simulink model "twoPhaseStickmanRev2022a"  (R2022a)
settings: Solver=VariableStepAuto  StartTime=0.0  StopTime=10  RelTol=1e-3
libraries: aerolibanim x1, shared6dof x1
settings Model: Creator=matho  LastModifiedBy=matho
settings ModelReferenceCC: EnableRefExpFcnMdlSchedulingChecks=off
settings RTWCC: Description=Generic Real-Time Target

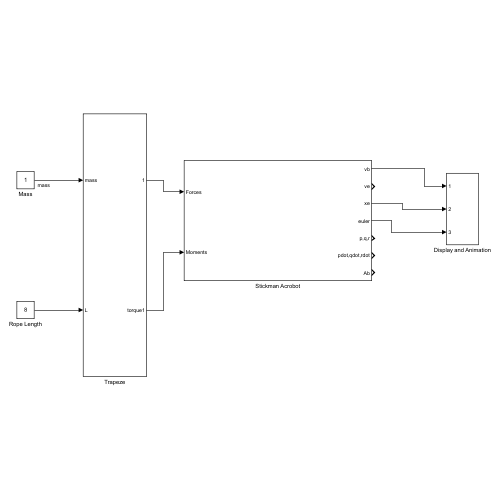
[thumbnail: Simulink's stored preview of the top-level diagram]
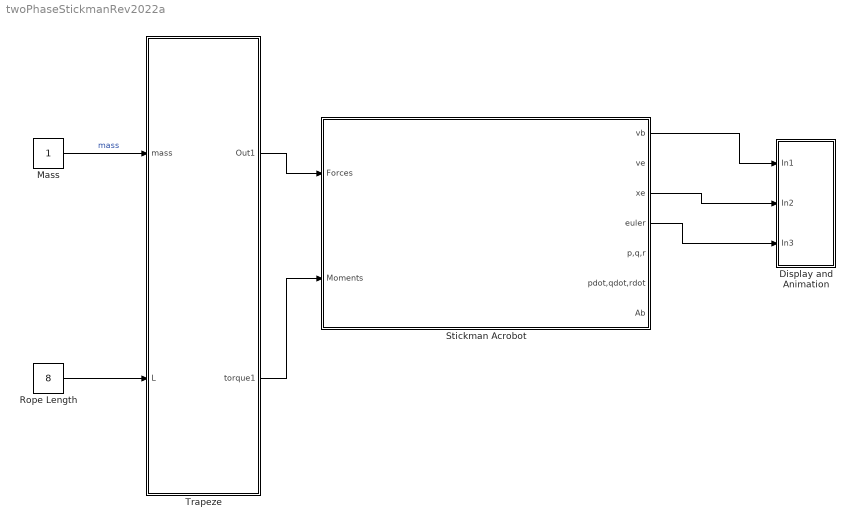
== system twoPhaseStickmanRev2022a ==
  Display and Animation : Subsystem
  Mass : Constant
  Rope Length : Constant  Value=8
  Stickman Acrobot : Subsystem
  Trapeze : Subsystem
  wires:
  Mass/1 -> Trapeze/1(mass)  "mass"
  Rope Length/1 -> Trapeze/2(L)
  Trapeze/1(Out1) -> Stickman Acrobot/1(Forces)
  Trapeze/2(torque1) -> Stickman Acrobot/2(Moments)
  Stickman Acrobot/1(vb) -> Display and Animation/1(In1)
  Stickman Acrobot/3(xe) -> Display and Animation/2(In2)
  Stickman Acrobot/4(euler) -> Display and Animation/3(In3)

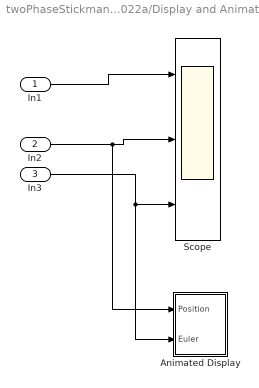
== system twoPhaseStickmanRev2022a/Display and Animation ==
  In1 : Inport
  In2 : Inport  Port=2
  In3 : Inport  Port=3
  Animated Display : Subsystem
  Scope : Scope  NumInputPorts=3
  wires:
  In2/1 -> Animated Display/1(Position), Scope/2
  In3/1 -> Animated Display/2(Euler), Scope/3
  In1/1 -> Scope/1

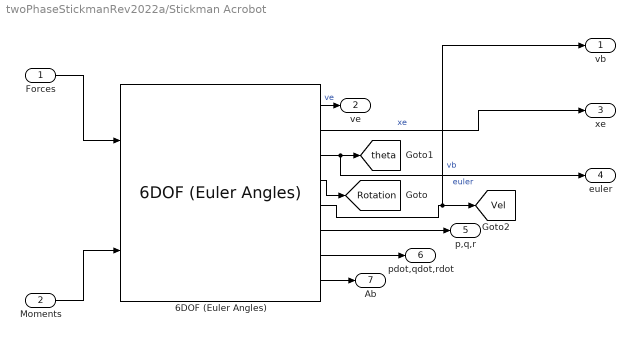
== system twoPhaseStickmanRev2022a/Stickman Acrobot ==
  Forces : Inport
  Moments : Inport  Port=2
  6DOF (Euler Angles) : shared6dof/6DOF (Euler Angles)  units=Metric (MKS)  mtype=Fixed  rep=Euler Angles  xme_0=[-8 0 -8]  Vm_0=[0 0 0]  eul_0=[0 -1.5 0]  pm_0=[0 0 0]  mass_0=1.0  mass_e=0.5  mass_f=2.0  inertia=eye(3)  inertia_e=eye(3)  inertia_f=2*eye(3)  k_quat=1.0  vre_flag=on  abi_flag=off  aMode=0  xme_statename=''  Vm_statename=''  eul_statename=''  quat_statename=''  pm_statename=''  mass_statename=''
  vb : Outport
  ve : Outport  Port=2
  xe : Outport  Port=3
  euler : Outport  Port=4
  p,q,r : Outport  Port=5
  pdot,qdot,rdot : Outport  Port=6
  Ab : Outport  Port=7
  tag scope: Rotation=global, Vel=global, theta=global
  wires:
  Moments/1 -> 6DOF (Euler Angles)/2
  6DOF (Euler Angles)/5 -> vb/1, [Vel]  "vb"
  6DOF (Euler Angles)/3 -> euler/1, [theta]  "euler"
  6DOF (Euler Angles)/8 -> Ab/1
  6DOF (Euler Angles)/4 -> [Rotation]
  6DOF (Euler Angles)/2 -> xe/1  "xe"
  Forces/1 -> 6DOF (Euler Angles)/1
  6DOF (Euler Angles)/6 -> p,q,r/1
  6DOF (Euler Angles)/1 -> ve/1  "ve"
  6DOF (Euler Angles)/7 -> pdot,qdot,rdot/1

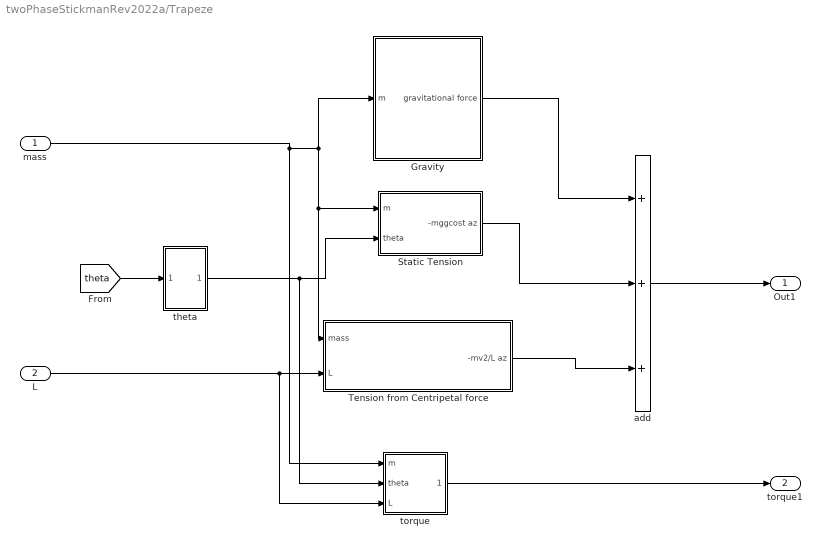
== system twoPhaseStickmanRev2022a/Trapeze ==
  mass : Inport
  L : Inport  Port=2
  Gravity : Subsystem
  Static Tension : Subsystem
  Tension from Centripetal force : Subsystem
  add : Sum  Inputs=+++
  theta : Subsystem
  torque : Subsystem
  Out1 : Outport
  torque1 : Outport  Port=2
  wires:
  theta/1(Out1) -> torque/2(theta), Static Tension/2(theta)
  [theta] -> theta/1(In1)
  mass/1 -> Tension from Centripetal force/1(mass), Static Tension/1(m), Gravity/1(m), torque/1(m)
  Tension from Centripetal force/1(-mv2/L az) -> add/3
  Static Tension/1(-mggcost az) -> add/2
  Gravity/1(gravitational force) -> add/1
  L/1 -> torque/3(L), Tension from Centripetal force/2(L)
  add/1 -> Out1/1
  torque/1(torque) -> torque1/1

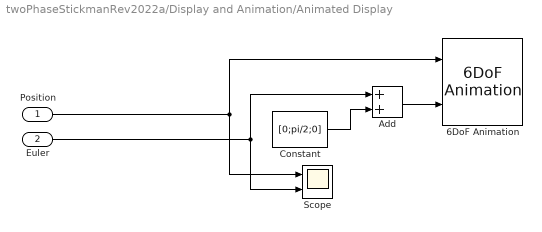
== system twoPhaseStickmanRev2022a/Display and Animation/Animated Display ==
  Position : Inport
  Euler : Inport  Port=2
  6DoF Animation : aerolibanim/6DoF Animation  u1=[-50 50 -50 50 -100 0]  u2=0.05  u3=3.0  u4=[0,0,0]  u5=Fixed position  u6=[10,10,0]  u7=90  u8=on
  Add : Sum
  Constant : Constant  Value=[0;pi/2;0]
  Scope : Scope  NumInputPorts=2
  wires:
  Euler/1 -> Add/1, Scope/2
  Position/1 -> Scope/1, 6DoF Animation/1
  Add/1 -> 6DoF Animation/2
  Constant/1 -> Add/2

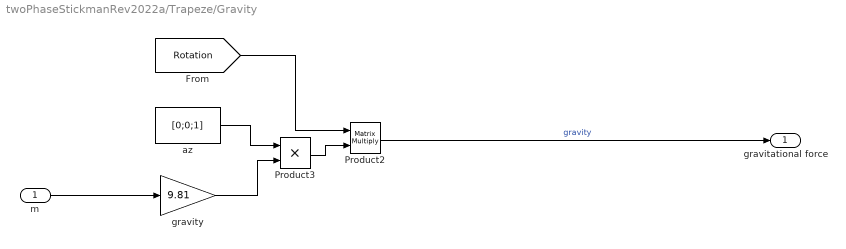
== system twoPhaseStickmanRev2022a/Trapeze/Gravity ==
  m : Inport
  Product2 : Product  Multiplication=Matrix(*)
  Product3 : Product
  az : Constant  Value=[0;0;1]
  gravity : Gain  Gain=9.81
  gravitational force : Outport
  wires:
  [Rotation] -> Product2/1
  az/1 -> Product3/1
  gravity/1 -> Product3/2
  Product3/1 -> Product2/2
  Product2/1 -> gravitational force/1  "gravity"
  m/1 -> gravity/1

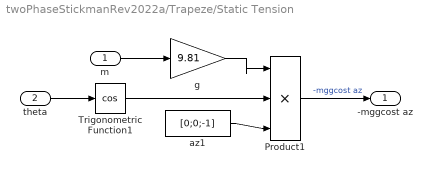
== system twoPhaseStickmanRev2022a/Trapeze/Static Tension ==
  m : Inport
  theta : Inport  Port=2
  Product1 : Product  Inputs=3
  Trigonometric Function1 : Trigonometry  Operator=cos
  az1 : Constant  Value=[0;0;-1]
  g : Gain  Gain=9.81
  -mggcost az : Outport
  wires:
  m/1 -> g/1
  az1/1 -> Product1/3
  Trigonometric Function1/1 -> Product1/2
  g/1 -> Product1/1
  theta/1 -> Trigonometric Function1/1
  Product1/1 -> -mggcost az/1  "-mggcost az"

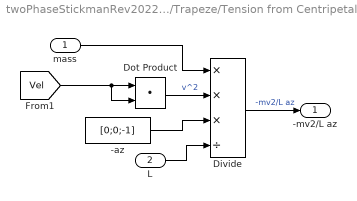
== system twoPhaseStickmanRev2022a/Trapeze/Tension from Centripetal force ==
  mass : Inport
  L : Inport  Port=2
  -az : Constant  Value=[0;0;-1]
  Divide : Product  Inputs=***/
  Dot Product : DotProduct  OutDataTypeStr=Inherit: Inherit via internal rule
  -mv2/L az : Outport
  wires:
  -az/1 -> Divide/3
  [Vel] -> Dot Product/2, Dot Product/1
  Dot Product/1 -> Divide/2  "v^2"
  L/1 -> Divide/4
  Divide/1 -> -mv2/L az/1  "-mv2/L az"
  mass/1 -> Divide/1

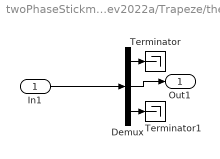
== system twoPhaseStickmanRev2022a/Trapeze/theta ==
  In1 : Inport
  Demux : Demux  Outputs=3
  Terminator : Terminator
  Terminator1 : Terminator
  Out1 : Outport
  wires:
  Demux/3 -> Terminator1/1
  Demux/1 -> Terminator/1
  Demux/2 -> Out1/1
  In1/1 -> Demux/1

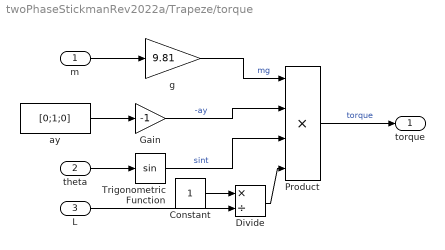
== system twoPhaseStickmanRev2022a/Trapeze/torque ==
  m : Inport
  theta : Inport  Port=2
  L : Inport  Port=3
  Constant : Constant
  Divide : Product  Inputs=*/
  Gain : Gain  Gain=-1
  Product : Product  Inputs=4
  Trigonometric Function : Trigonometry
  ay : Constant  Value=[0;1;0]
  g : Gain  Gain=9.81
  torque : Outport
  wires:
  theta/1 -> Trigonometric Function/1
  L/1 -> Divide/2
  g/1 -> Product/1  "mg"
  ay/1 -> Gain/1
  Gain/1 -> Product/2  "-ay"
  Trigonometric Function/1 -> Product/3  "sint"
  m/1 -> g/1
  Product/1 -> torque/1  "torque"
  Constant/1 -> Divide/1
  Divide/1 -> Product/4
